simulink model "EZQ4sFlow"  (R2018b)
settings: Solver=FixedStepDiscrete  StartTime=0.0  StopTime=10.0  FixedStep=0.01  RelTol=1e-3
settings Model: ModifiedHistory=2023.8.1 V2.0.0 CR421790 增加模式21-26  Creator=sn2xws  LastModifiedBy=sn2xws
settings DataIOCC: SaveFormat=StructureWithTime
settings OptimizationCC: DefaultParameterBehavior=Inlined  EnhancedBackFolding=on  PassReuseOutputArgsAs=Individual arguments  ZeroExternalMemoryAtStartup=off  ZeroInternalMemoryAtStartup=off  OptimizeBlockOrder=speed  DifferentSizesBufferReuse=on  OptimizationCustomize=off
settings DebuggingCC: ParameterTunabilityLossMsg=error
settings SFSimCC: MATLABDynamicMemAlloc=off
settings RTWCC: SystemTargetFile=autosar.tlc  GenCodeOnly=on  TemplateMakefile=ert_default_tmf  Description=AUTOSAR  GenerateReport=on  IncludeHyperlinkInReport=on  LaunchReport=on  GenerateTraceInfo=on  GenerateTraceReport=on  GenerateTraceReportSl=on  GenerateTraceReportSf=on  GenerateTraceReportEml=on  GenerateCodeMetricsReport=on
settings CodeAppCC: ForceParamTrailComments=on  IgnoreCustomStorageClasses=off  OperatorAnnotations=on  SimulinkDataObjDesc=on  SFDataObjDesc=on  InsertBlockDesc=on
settings STFCustomTargetCC: TargetLangStandard=C99 (ISO)  MultiwordLength=256  ParMdlRefBuildCompliant=on  CompOptLevelCompliant=on  IncludeMdlTerminateFcn=off  CombineOutputUpdateFcns=on  SuppressErrorStatus=on  ERTCustomFileBanners=on  SupportNonFinite=off  SupportComplex=off  SupportContinuousTime=off  SupportNonInlinedSFcns=off  RemoveResetFunc=on  MATLABClassNameForMDSCustomization=Simulink.SoftwareTarget.ERTCustomization  AutosarCompliant=on  UseToolchainInfoCompliant=on  LookupTableObjectStructAxisOrder=2,1,3,4,...  LUTObjectStructOrderEvenSpacing=Size,Table,Breakpoints  SystemTargetFile=autosar.tlc
settings ERTTargetCC: TargetLangStandard=C99 (ISO)  ConcurrentExecutionCompliant=off  IncludeMdlTerminateFcn=off  SuppressErrorStatus=on  SupportNonFinite=off  SupportComplex=off  ModelStepFunctionPrototypeControlCompliant=off  CPPClassGenCompliant=off  AutosarCompliant=on  LookupTableObjectStructAxisOrder=2,1,3,4,...  LUTObjectStructOrderEvenSpacing=Size,Table,Breakpoints  InlinedParameterPlacement=NonHierarchical  ERTCustomFileTemplate=example_file_process.tlc  ERTFilePackagingFormat=Compact

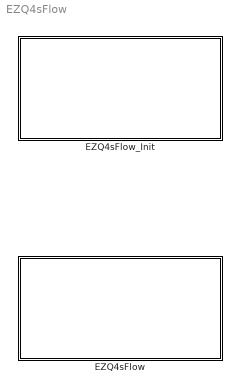
== system EZQ4sFlow ==
  EZQ4sFlow : Subsystem
  EZQ4sFlow_Init : Subsystem

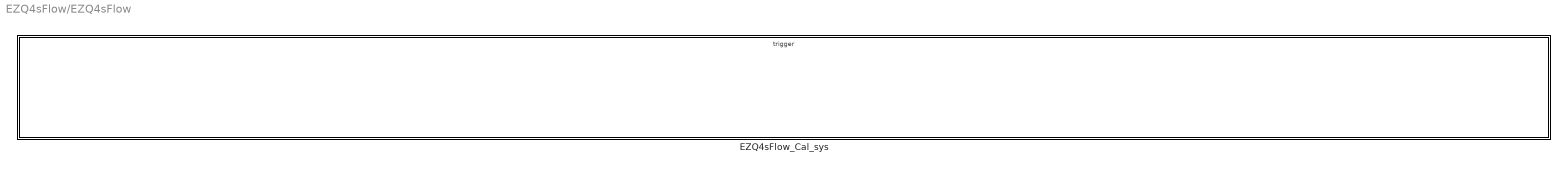
== system EZQ4sFlow/EZQ4sFlow ==
  EZQ4sFlow_Cal_sys : Subsystem

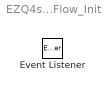
== system EZQ4sFlow/EZQ4sFlow_Init ==
  Event Listener : EventListener  EventName=reset

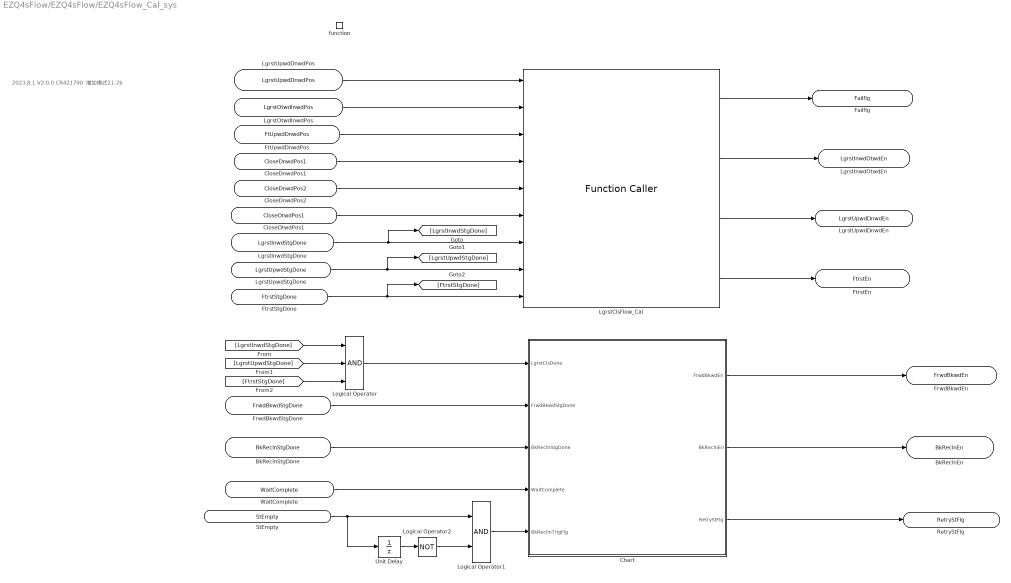
== system EZQ4sFlow/EZQ4sFlow/EZQ4sFlow_Cal_sys ==
  note: 2023.8.1 V2.0.0 CR421790 增加模式21-26
  function : TriggerPort  TriggerType=function-call  IsSimulinkFunction=on  FunctionName=EZQ4sFlow_Cal  VariantControl=(inherit)
  Chart : Stateflow chart  TreatAsAtomicUnit=on
  LgrstClsFlow_Cal : FunctionCaller  FunctionPrototype=[Failflg,LgrstInwdOtwdEn,LgrstUpwdDnwdEn,FtrstEn] = LgrstClsFlow_Cal(LgrstUpwdDnwdPos,LgrstOtwdInwdPos,FtUpwdDnwdPos,CloseDnwdPos1,CloseDnwdPos2,CloseOtwdPos1,LgrstInwdStgDone,LgrstUpwdStgDone,FtrstStgDone)  InputArgumentSpecifications=uint16(1), uint16(1), uint16(1), uint16(1), uint16(1), uint16(1), boolean(true), boolean(true), boolean(true)  OutputArgumentSpecifications=boolean(true), boolean(true), boolean(true), boolean(true)
  Logical Operator : Logic  Inputs=3  AllPortsSameDT=off  OutDataTypeStr=boolean
  Logical Operator1 : Logic  AllPortsSameDT=off  OutDataTypeStr=boolean
  Logical Operator2 : Logic  Operator=NOT  AllPortsSameDT=off  OutDataTypeStr=boolean
  Unit Delay : UnitDelay  InitialCondition=1  SampleTime=-1
  LgrstUpwdDnwdPos : ArgIn  OutDataTypeStr=uint16  ArgumentName=LgrstUpwdDnwdPos
  LgrstOtwdInwdPos : ArgIn  Port=2  OutDataTypeStr=uint16  ArgumentName=LgrstOtwdInwdPos
  FtUpwdDnwdPos : ArgIn  Port=3  OutDataTypeStr=uint16  ArgumentName=FtUpwdDnwdPos
  CloseDnwdPos1 : ArgIn  Port=4  OutDataTypeStr=uint16  ArgumentName=CloseDnwdPos1
  CloseDnwdPos2 : ArgIn  Port=5  OutDataTypeStr=uint16  ArgumentName=CloseDnwdPos2
  CloseOtwdPos1 : ArgIn  Port=6  OutDataTypeStr=uint16  ArgumentName=CloseOtwdPos1
  LgrstInwdStgDone : ArgIn  Port=7  OutDataTypeStr=boolean  ArgumentName=LgrstInwdStgDone
  LgrstUpwdStgDone : ArgIn  Port=8  OutDataTypeStr=boolean  ArgumentName=LgrstUpwdStgDone
  FtrstStgDone : ArgIn  Port=9  OutDataTypeStr=boolean  ArgumentName=FtrstStgDone
  FrwdBkwdStgDone : ArgIn  Port=10  OutDataTypeStr=boolean  ArgumentName=FrwdBkwdStgDone
  BkReclnStgDone : ArgIn  Port=11  OutDataTypeStr=boolean  ArgumentName=BkReclnStgDone
  StEmpty : ArgIn  Port=12  OutDataTypeStr=boolean  ArgumentName=StEmpty
  WaitComplete : ArgIn  Port=13  OutDataTypeStr=boolean  ArgumentName=WaitComplete
  Failflg : ArgOut  OutDataTypeStr=boolean  ArgumentName=Failflg
  LgrstInwdOtwdEn : ArgOut  Port=2  OutDataTypeStr=boolean  ArgumentName=LgrstInwdOtwdEn
  LgrstUpwdDnwdEn : ArgOut  Port=3  OutDataTypeStr=boolean  ArgumentName=LgrstUpwdDnwdEn
  FtrstEn : ArgOut  Port=4  OutDataTypeStr=boolean  ArgumentName=FtrstEn
  FrwdBkwdEn : ArgOut  Port=5  OutDataTypeStr=boolean  ArgumentName=FrwdBkwdEn
  BkReclnEn : ArgOut  Port=6  OutDataTypeStr=boolean  ArgumentName=BkReclnEn
  RetryStFlg : ArgOut  Port=7  OutDataTypeStr=boolean  ArgumentName=RetryStFlg
  wires:
  LgrstClsFlow_Cal/1 -> Failflg/1
  LgrstClsFlow_Cal/2 -> LgrstInwdOtwdEn/1
  LgrstClsFlow_Cal/3 -> LgrstUpwdDnwdEn/1
  LgrstClsFlow_Cal/4 -> FtrstEn/1
  LgrstUpwdDnwdPos/1 -> LgrstClsFlow_Cal/1
  LgrstOtwdInwdPos/1 -> LgrstClsFlow_Cal/2
  FtUpwdDnwdPos/1 -> LgrstClsFlow_Cal/3
  CloseDnwdPos1/1 -> LgrstClsFlow_Cal/4
  CloseDnwdPos2/1 -> LgrstClsFlow_Cal/5
  CloseOtwdPos1/1 -> LgrstClsFlow_Cal/6
  LgrstInwdStgDone/1 -> [LgrstInwdStgDone], LgrstClsFlow_Cal/7
  LgrstUpwdStgDone/1 -> [LgrstUpwdStgDone], LgrstClsFlow_Cal/8
  FtrstStgDone/1 -> [FtrstStgDone], LgrstClsFlow_Cal/9
  [FtrstStgDone] -> Logical Operator/3
  [LgrstInwdStgDone] -> Logical Operator/1
  [LgrstUpwdStgDone] -> Logical Operator/2
  Logical Operator/1 -> Chart/1(LgrstClsDone)
  FrwdBkwdStgDone/1 -> Chart/2(FrwdBkwdStgDone)
  BkReclnStgDone/1 -> Chart/3(BkReclnStgDone)
  StEmpty/1 -> Unit Delay/1, Logical Operator1/1
  Chart/1(FrwdBkwdEn) -> FrwdBkwdEn/1
  Chart/2(BkReclnEn) -> BkReclnEn/1
  Logical Operator1/1 -> Chart/5(BkReclinTrigFlg)
  WaitComplete/1 -> Chart/4(WaitComplete)
  Chart/3(RetryStFlg) -> RetryStFlg/1
  Unit Delay/1 -> Logical Operator2/1
  Logical Operator2/1 -> Logical Operator1/2

== stateflow chart EZQ4sFlow/EZQ4sFlow_Cal_sys/Chart ==
  (default) -> (junction 8) : {
      | FrwdBkwdEn = 0;
      | BkReclnEn = 0;
      | RetryStFlg=0;
      | }
  (junction 8) -> (junction 10) [order 1] : [LgrstClsDone&&!FrwdBkwdStgDone]
  (junction 8) -> (junction 14) [order 2]
  (junction 10) -> (junction 12) : {FrwdBkwdEn=1;}
  (junction 12) -> (junction 14)
  (junction 14) -> (junction 18)
  (junction 18) -> (junction 20) [order 1] : [LgrstClsDone && FrwdBkwdStgDone&&!BkReclnStgDone]
  (junction 18) -> (junction 24) [order 2]
  (junction 20) -> (junction 22) : {BkReclnEn=1;}
  (junction 22) -> (junction 24)
  (junction 24) -> (junction 27)
  (junction 27) -> (junction 29) [order 1] : [!WaitComplete&&LgrstClsDone&&FrwdBkwdStgDone&&BkReclnStgDone]
  (junction 29) -> (junction 38) [order 1] : [BkReclinTrigFlg]
  (junction 27) -> (junction 36) [order 2]
  (junction 29) -> (junction 45) [order 2]
  (junction 38) -> (junction 42) : {
      | RetryStFlg=1;
      | }
  (junction 45) -> (junction 36)
  (junction 42) -> (junction 45)
  (junction 36) -> (junction 47)
  data: LgrstClsDone input; FrwdBkwdStgDone input; BkReclnStgDone input; FrwdBkwdEn output boolean; BkReclnEn output boolean; RetryStFlg output boolean; WaitComplete input boolean; BkReclinTrigFlg input boolean
